simulink model "part_3_sim"  (R2022b)
settings: Solver=ode4  StartTime=0.0  StopTime=10.0  FixedStep=0.001  RelTol=1e-3
values from neighbouring files (symbols this model uses):
  K = 20    [prob1.m]
  T = 1 / sample_rate    (= 0.1)    [p1.m]    (also in prob1.m = 0.25)
undefined symbols (not defined in the file or in its folder): p1, sat, z1
settings Model: Creator=bransoncamp  LastModifiedBy=bransoncamp

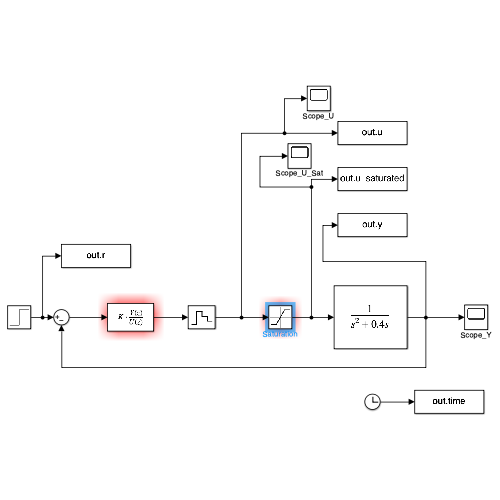
[thumbnail: Simulink's stored preview of the top-level diagram]
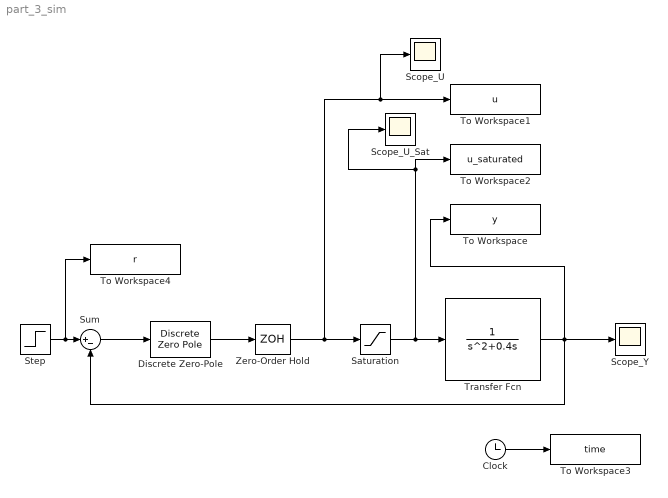
== system part_3_sim ==
  Clock : Clock
  Discrete Zero-Pole : DiscreteZeroPole  Zeros=z1  Poles=p1  Gain=K  SampleTime=T
  Saturation : Saturate  UpperLimit=sat  LowerLimit=-sat
  Scope_U : Scope
  Scope_U_Sat : Scope
  Scope_Y : Scope
  Step : Step  SampleTime=0
  Sum : Sum  Inputs=|+-
  To Workspace : ToWorkspace  VariableName=y  SaveFormat=Structure With Time  SampleTime=-1
  To Workspace1 : ToWorkspace  VariableName=u  SaveFormat=Structure With Time  SampleTime=-1
  To Workspace2 : ToWorkspace  VariableName=u_saturated  SaveFormat=Structure With Time  SampleTime=-1
  To Workspace3 : ToWorkspace  VariableName=time  SampleTime=-1
      settings: Decimation=3
  To Workspace4 : ToWorkspace  VariableName=r  SaveFormat=Structure With Time  SampleTime=-1
  Transfer Fcn : TransferFcn  Denominator=[1 0.4 0]
  Zero-Order Hold : ZeroOrderHold  SampleTime=-1
  wires:
  Saturation/1 -> Scope_U_Sat/1, To Workspace2/1, Transfer Fcn/1
  Zero-Order Hold/1 -> Scope_U/1, To Workspace1/1, Saturation/1
  Sum/1 -> Discrete Zero-Pole/1
  Discrete Zero-Pole/1 -> Zero-Order Hold/1
  Transfer Fcn/1 -> Scope_Y/1, To Workspace/1, Sum/2
  Step/1 -> To Workspace4/1, Sum/1
  Clock/1 -> To Workspace3/1
